simulink model "Sim_AdaptivePlanta_ultimo"  (R2016a)
settings: Solver=ode45  StartTime=0.0  StopTime=20  FixedStep=0.01  MaxStep=0.01  RelTol=1e-3
values from neighbouring files (symbols this model uses):
  b = [0;1]    [parametros_ultimo.m]
  g = 9.8    [parametros_ultimo.m]
  J = 42.51    [parametros_ultimo.m]
  k = 0.14893    [parametros_ultimo.m]
  Kd = 10000    [leyDeControl.m]    (also in parametros_ultimo.m)
  Kp = 100000    [leyDeControl.m]    (also in parametros_ultimo.m)
  l = 0.05    [parametros_ultimo.m]
  P = lyap(A,Q)    [leyDeControl.m]    (also in parametros_ultimo.m = lyap(a,0.2*eye(2)))
  R = 6    [parametros_ultimo.m]
settings Model: Creator=Harryth  LastModifiedBy=i95sa
settings DataIOCC: LimitDataPoints=on  SaveFormat=Array  SignalLoggingSaveFormat=ModelDataLogs
settings OptimizationCC: ExpressionDepthLimit=2147483647
settings DebuggingCC: UnderspecifiedInitializationDetection=Classic  MergeDetectMultiDrivingBlocksExec=none  SolverPrmCheckMsg=warning  FcnCallInpInsideContextMsg=UseLocalSettings  StateNameClashWarn=warning
settings HardwareCC: ProdBitPerPointer=32  ProdLargestAtomicFloat=None  ProdIntDivRoundTo=Undefined  ProdEndianess=Unspecified  ProdWordSize=32  ProdHWDeviceType=32-bit Generic
settings ModelReferenceCC: PropagateSignalLabelsOutOfModel=off
settings GRTTargetCC: CombineOutputUpdateFcns=off  GRTInterface=on
settings ConfigComp: CovModelRefEnable=Off

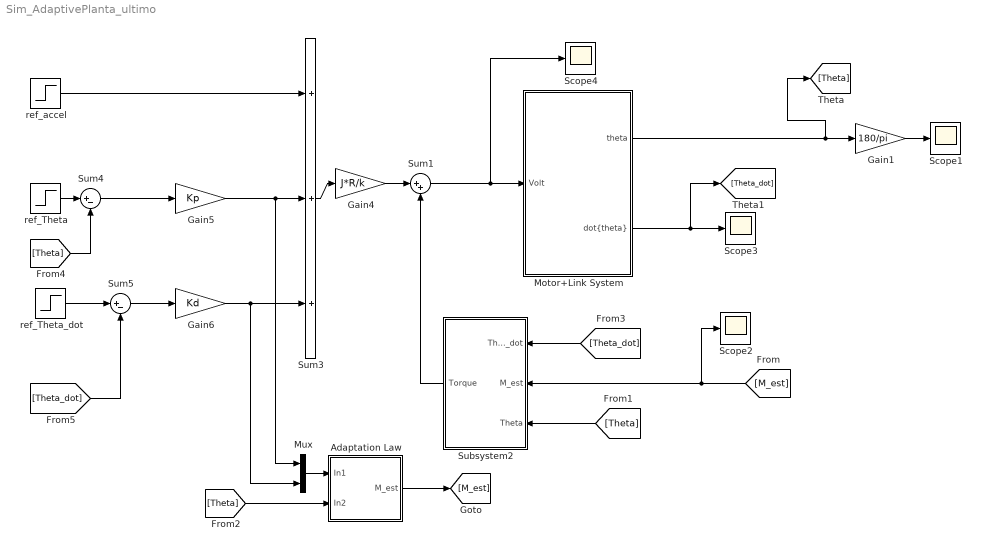
== system Sim_AdaptivePlanta_ultimo ==
  Adaptation Law : Subsystem
  Gain1 : Gain  Gain=180/pi
  Gain4 : Gain  Gain=J*R/k
  Gain5 : Gain  Gain=Kp
  Gain6 : Gain  Gain=Kd
  Motor+Link System : Subsystem
  Mux : Mux  Inputs=2
  Scope{1..4} (4 alike) : Scope
  Subsystem2 : Subsystem
  Sum1 : Sum  Inputs=|++
  Sum3 : Sum  Inputs=+++
  Sum4 : Sum  Inputs=|+-
  Sum5 : Sum  Inputs=|+-
  ref_Theta : Step  SampleTime=0
  ref_Theta_dot : Step  After=0  SampleTime=0
  ref_accel : Step  After=0  SampleTime=0
  wires:
  Motor+Link System/1(theta) -> Gain1/1, [Theta]
  Motor+Link System/2("dot{theta}") -> Scope3/1, [Theta_dot]
  Sum1/1 -> Motor+Link System/1(Volt), Scope4/1
  Subsystem2/1(Torque) -> Sum1/2
  Gain4/1 -> Sum1/1
  Sum3/1 -> Gain4/1
  ref_accel/1 -> Sum3/1
  Sum4/1 -> Gain5/1
  Gain5/1 -> Sum3/2, Mux/1
  Sum5/1 -> Gain6/1
  Gain6/1 -> Sum3/3, Mux/2
  ref_Theta/1 -> Sum4/1
  ref_Theta_dot/1 -> Sum5/1
  Mux/1 -> Adaptation Law/1(In1)
  Adaptation Law/1(M_est) -> [M_est]
  [M_est] -> Scope2/1, Subsystem2/2(M_est)
  [Theta] -> Subsystem2/3(Theta)
  [Theta] -> Adaptation Law/2(In2)
  [Theta_dot] -> Subsystem2/1(Theta_dot)
  [Theta] -> Sum4/2
  [Theta_dot] -> Sum5/2
  Gain1/1 -> Scope1/1

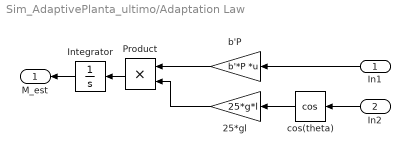
== system Sim_AdaptivePlanta_ultimo/Adaptation Law ==
  In1 : Inport
  In2 : Inport  Port=2
  25*gl : Gain  Gain=25*g*l
  Integrator : Integrator  InitialCondition=50
  Product : Product  RndMeth=Zero
  b'P : Gain  Gain=b'*P  Multiplication=Matrix(K*u) (u vector)
  cos(theta) : Trigonometry  Operator=cos
  M_est : Outport
  wires:
  cos(theta)/1 -> 25*gl/1
  25*gl/1 -> Product/2
  Integrator/1 -> M_est/1
  In2/1 -> cos(theta)/1
  Product/1 -> Integrator/1
  In1/1 -> b'P/1
  b'P/1 -> Product/1

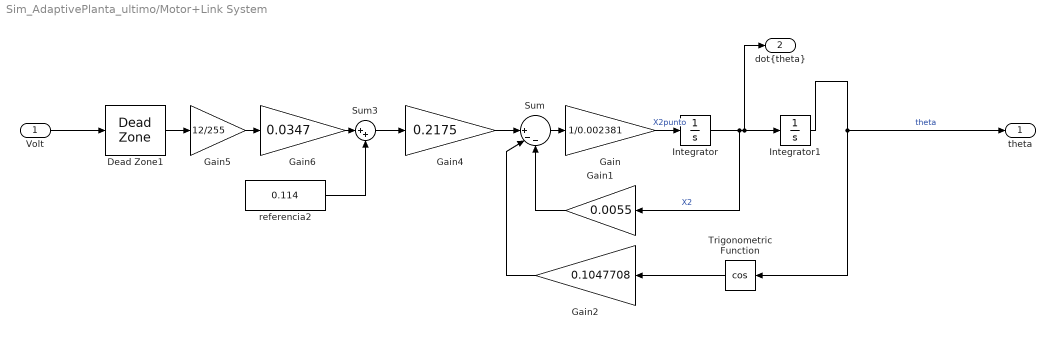
== system Sim_AdaptivePlanta_ultimo/Motor+Link System ==
  Volt : Inport
  Dead Zone1 : DeadZone  LowerValue=0  UpperValue=0  SaturateOnIntegerOverflow=on
  Gain : Gain  Gain=1/0.002381
  Gain1 : Gain  Gain=0.0055
  Gain2 : Gain  Gain=0.1047708
  Gain4 : Gain  Gain=0.2175
  Gain5 : Gain  Gain=12/255
  Gain6 : Gain  Gain=0.0347
  Integrator : Integrator
  Integrator1 : Integrator  InitialCondition=-0.65
  Sum : Sum  Inputs=||+--
  Sum3 : Sum  Inputs=|++
  Trigonometric Function : Trigonometry  Operator=cos
  referencia2 : Constant  Value=0.114
  theta : Outport
  "dot{theta}" : Outport  Port=2
  wires:
  Sum/1 -> Gain/1
  Gain/1 -> Integrator/1  "X2punto"
  Integrator/1 -> "dot{theta}"/1, Integrator1/1, Gain1/1  "X2"
  Trigonometric Function/1 -> Gain2/1
  Gain1/1 -> Sum/3
  Integrator1/1 -> theta/1, Trigonometric Function/1  "theta"
  Gain2/1 -> Sum/2
  Gain4/1 -> Sum/1
  referencia2/1 -> Sum3/2
  Sum3/1 -> Gain4/1
  Gain5/1 -> Gain6/1
  Gain6/1 -> Sum3/1
  Dead Zone1/1 -> Gain5/1
  Volt/1 -> Dead Zone1/1

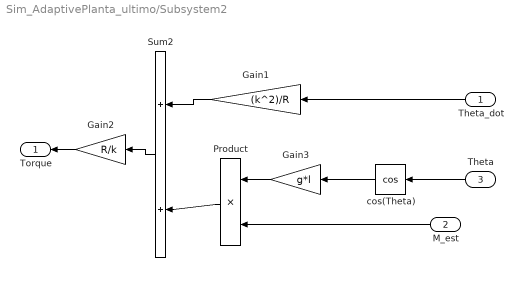
== system Sim_AdaptivePlanta_ultimo/Subsystem2 ==
  Theta_dot : Inport
  M_est : Inport  Port=2
  Theta : Inport  Port=3
  Gain1 : Gain  Gain=(k^2)/R
  Gain2 : Gain  Gain=R/k
  Gain3 : Gain  Gain=g*l
  Product : Product  RndMeth=Zero
  Sum2 : Sum
  cos(Theta) : Trigonometry  Operator=cos
  Torque : Outport
  wires:
  cos(Theta)/1 -> Gain3/1
  Sum2/1 -> Gain2/1
  Gain1/1 -> Sum2/1
  Gain3/1 -> Product/1
  Product/1 -> Sum2/2
  Theta_dot/1 -> Gain1/1
  Theta/1 -> cos(Theta)/1
  Gain2/1 -> Torque/1
  M_est/1 -> Product/2
